simulink model "delta_modulation"  (R2022b)
settings: Solver=VariableStepAuto  StartTime=0.0  StopTime=2  RelTol=1e-3
libraries: dspquant2 x2, dsparch4 x1
settings Model: Creator=Admin  LastModifiedBy=Aman
settings SolverCC: AlgebraicLoopSolver=TrustRegion
settings DataIOCC: ReturnWorkspaceOutputs=off
settings DebuggingCC: UnconnectedInputMsg=warning  UnconnectedOutputMsg=warning  UnconnectedLineMsg=warning  SFMachineParentedDataDiag=warning  ArithmeticOperatorsInVariantConditions=warning
settings ModelReferenceCC: EnableRefExpFcnMdlSchedulingChecks=on
settings SFSimCC: CustomCodeUndefinedFunction=UseInterfaceOnly

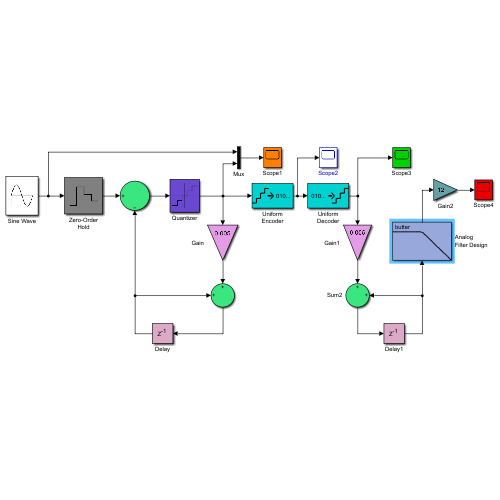
[thumbnail: Simulink's stored preview of the top-level diagram]
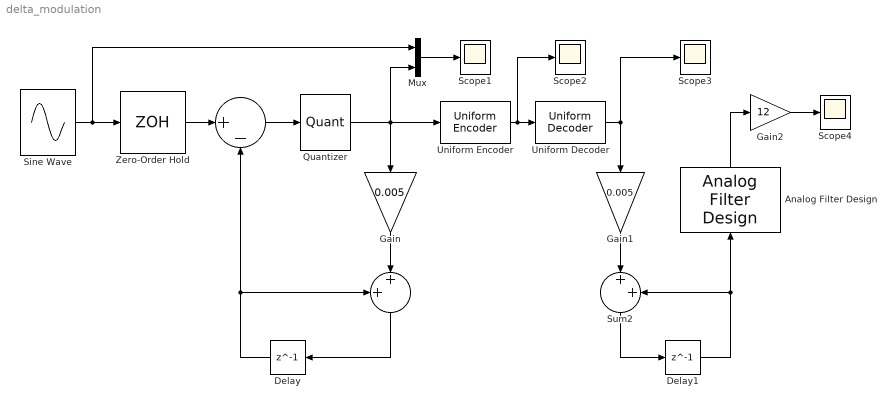
== system delta_modulation ==
  " " : Sum  Inputs=|+-
  " " : Sum  Inputs=++|
  "     Sum2" : Sum  Inputs=|++
  Analog Filter Design : dsparch4/Analog Filter Design  method=Butterworth  filttype=Lowpass  N=8  Wlo=2*pi*100  Whi=80  Rp=2  Rs=40
  Delay : Delay  DelayLength=1  InitialCondition=0
  Delay1 : Delay  DelayLength=1  InitialCondition=0
  Gain : Gain  Gain=0.005
  Gain1 : Gain  Gain=0.005
  Gain2 : Gain  Gain=12
  Mux : Mux  Inputs=2
  Quantizer : Quantizer
  Scope1 : Scope
  "Scope2 " : Scope
  "Scope3 " : Scope
  "Scope4 " : Scope
  Sine Wave : Sin  Amplitude=1.5  Frequency=2 *pi* 80  Samples=1000  SampleTime=0
  Uniform Decoder : dspquant2/Uniform Decoder  peak=2  bits=8  overflowMode=Saturate  otype=Double
  Uniform Encoder : dspquant2/Uniform Encoder  peak=2  bits=8  otype=Signed integer
  Zero-Order Hold : ZeroOrderHold  SampleTime=1/8000
  wires:
  Sine Wave/1 -> Mux/1, Zero-Order Hold/1
  Delay/1 -> " "/1, " "/2
  " "/1 -> Quantizer/1
  Quantizer/1 -> Mux/2, Uniform Encoder/1, Gain/1
  Mux/1 -> Scope1/1
  Zero-Order Hold/1 -> " "/1
  " "/1 -> Delay/1
  Gain1/1 -> "     Sum2"/1
  "     Sum2"/1 -> Delay1/1
  Delay1/1 -> Analog Filter Design/1, "     Sum2"/2
  Analog Filter Design/1 -> Gain2/1
  Gain2/1 -> "Scope4 "/1
  Uniform Decoder/1 -> "Scope3 "/1, Gain1/1
  Gain/1 -> " "/2
  Uniform Encoder/1 -> "Scope2 "/1, Uniform Decoder/1
